simulink model "simulink_template_2"  (R2024b)
settings: Solver=VariableStepAuto  StartTime=0.0  StopTime=T_SIMULATION  RelTol=1e-3
undefined symbols (not defined in the file or in its folder): d, OMEGA_L, OMEGA_R, Q_INITIAL, r
settings Model: Creator=alber  LastModifiedBy=Enrico

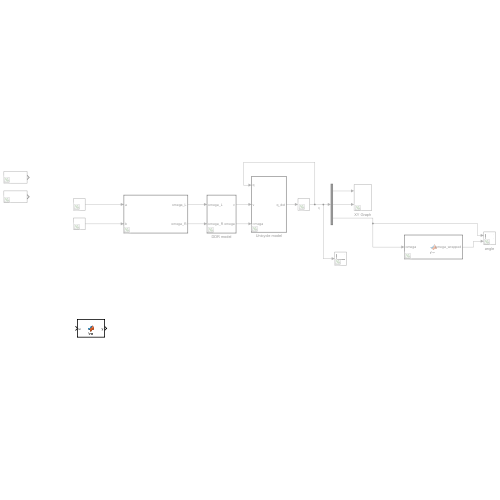
[thumbnail: Simulink's stored preview of the top-level diagram]
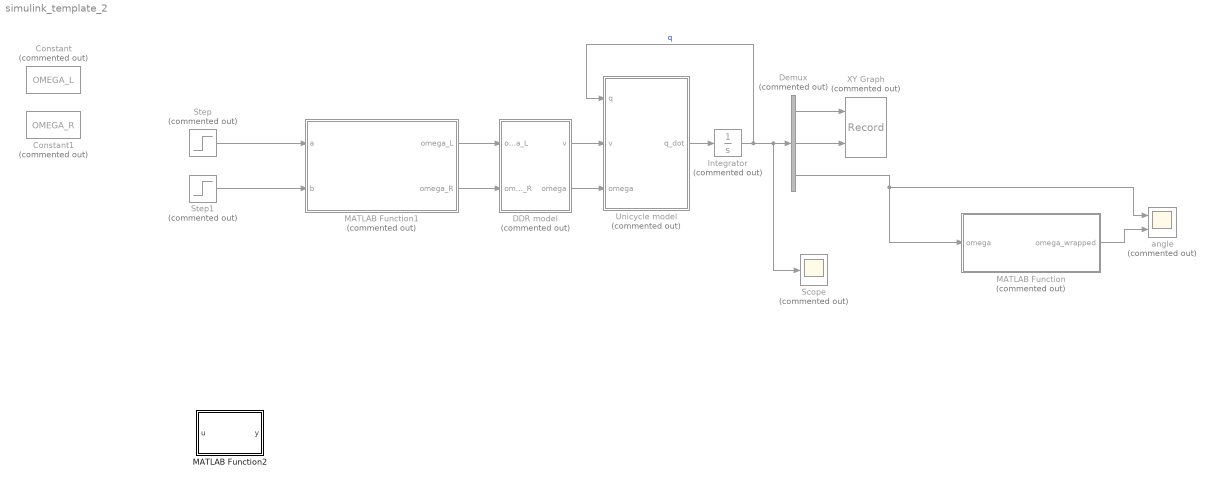
== system simulink_template_2 ==
  Constant : Constant  Commented=on  Value=OMEGA_L
  Constant1 : Constant  Commented=on  Value=OMEGA_R
  DDR model : MATLAB Function  Commented=on  TreatAsAtomicUnit=on
  Demux : Demux  Commented=on  Outputs=3
  Integrator : Integrator  Commented=on  InitialCondition=Q_INITIAL
  MATLAB Function : MATLAB Function  Commented=on  TreatAsAtomicUnit=on
  MATLAB Function1 : MATLAB Function  Commented=on  TreatAsAtomicUnit=on
  MATLAB Function2 : MATLAB Function  TreatAsAtomicUnit=on
  Scope : Scope  Commented=on
  Step : Step  Commented=on  SampleTime=0
  Step1 : Step  Commented=on  After=20  SampleTime=0
  Unicycle model : MATLAB Function  Commented=on  TreatAsAtomicUnit=on
  XY Graph : Record  Commented=on  FileSettingsInternal="{\"entries\":[{\"content\":{\"excelSettings\":{\"content\":{},\"type\":\"Streamout.ExcelSettings\"}},\"type\":\"Streamout.FileSettingStorage\",\"uuid\":\"\"}],\"packageUris\":[\"http:\\/\\/schema.mathworks.com\\/mf0\\/streamout_blocks\\/R2020a\"],\"version\":\"1.0\"}"  Layout=[1 1]  SignalsInternal="{\"entries\":[{\"content\":{},\"type\":\"RecordBlkView.InputSignals\",\"uuid\":\"\"}],\"packageUris\":[\"http:\\/\\/schema.mathworks.com\\/mf0\\/streamout_blocks\\/R2020a\"],\"version\":\"1.0\"}"  VisualizationBindings="{\"xyplotplugin\":{\"info\":[{\"series\":[],\"subplotID\":1}]}}"  CompatibilityTag=XY
  angle : Scope  Commented=on  NumInputPorts=2
  wires:
  Unicycle model/1(q_dot) -> Integrator/1
  DDR model/2(omega) -> Unicycle model/3(omega)
  DDR model/1(v) -> Unicycle model/2(v)
  Integrator/1 -> Scope/1, Demux/1, Unicycle model/1(q)  "q"
  Demux/2 -> XY Graph/2
  Demux/1 -> XY Graph/1
  MATLAB Function1/2(omega_R) -> DDR model/2(omega_R)
  MATLAB Function1/1(omega_L) -> DDR model/1(omega_L)
  Step/1 -> MATLAB Function1/1(a)
  Step1/1 -> MATLAB Function1/2(b)
  MATLAB Function/1(omega_wrapped) -> angle/2
  Demux/3 -> angle/1, MATLAB Function/1(omega)

== matlab function simulink_template_2/Unicycle model ==
  data: q input; v input; q_dot output; omega input; r parameter; d parameter
function q_dot = fcn(q, v, omega, r, d)
%write the unicycle model
%q_dot= zeros(3,1);
q_dot = [cos(q(3))*v; sin(q(3))*v; omega];

== matlab function simulink_template_2/DDR model ==
  data: omega_L input; v output; omega_R input; omega output; r parameter; d parameter
function [v, omega] = fcn(omega_L, omega_R, r, d)
%write the DDR model and return v and omega
v     = (r*omega_L + r*omega_R) / 2;
omega = (-r*omega_L + r*omega_R) / d;

== matlab function simulink_template_2/MATLAB Function ==
  data: omega input; omega_wrapped output
function omega_wrapped = fcn(omega)

omega_wrapped = wrapToPi(omega);

== matlab function simulink_template_2/MATLAB Function1 ==
  data: a input; omega_L output; b input; omega_R output
function [omega_L, omega_R]= fcn(a,b)

omega_L = a;
omega_R = b;

== matlab function simulink_template_2/MATLAB Function2 ==
  data: u input; y output
function y = fcn(u)
    % given initial and final config qi qf write a f that plan a traj form qi
    % to qf using the cart polyn strategy

    % can choose initial and final velocity
y = u;
